simulink model "s3_PMSG"  (R2019b)
settings: Solver=daessc  StartTime=0.0  StopTime=15  MinStep=1e-4  RelTol=1
libraries: powerlib x18, powerlib_meascontrol x2, simulink_extras x1
settings Model: SimulationMode=accelerator  Creator=MAHMUD  LastModifiedBy=MAHMUD

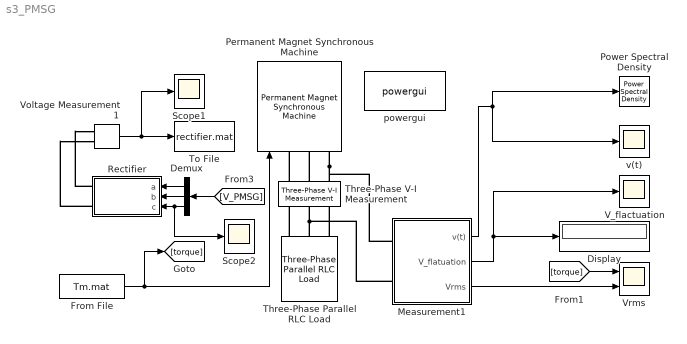
== system s3_PMSG ==
  Demux : Demux  Outputs=3
  Display : Display
  From File : FromFile  FileName=Tm.mat  SampleTime=0
  Measurement1 : Subsystem
  Permanent Magnet Synchronous Machine : powerlib/Machines/Permanent Magnet Synchronous Machine  NbPhases=3  FluxDistribution=Sinusoidal  RotorType=Salient-pole  MechanicalLoad=Torque Tm  PresetModel=No  ShowDetailedParameters=on  MeasurementBus=off  Resistance=0.03  Inductance=8.5e-3  dqInductances=[0.0415 0.015]  La=0.000835  MachineConstant=Voltage Constant (V_peak L-L / krpm)  Flux=0.55133  VoltageCst=100  TorqueCst=0.82699  Flat=120  Mechanical=[0.201 4.5 1]  PolePairs=4  InitialConditions=[0,0, 0,0]  InitialConditions5ph=[0 0 0 0 0 0]  RefAngle=Aligned with phase A axis (original Park)  IterativeDiscreteModel=Trapezoidal non iterative  TsBlock=-1  TsPowergui=0
  Power Spectral Density : simulink_extras/Additional Sinks/Power Spectral Density  npts=5000  fftpts=512  HowOften=500  sampleT=0.001
      settings: SourceProductName=Simulink  SourceProductBaseCode=SL
  Rectifier : Subsystem
  Scope1 : Scope
  Scope2 : Scope
  Three-Phase Parallel RLC Load : powerlib/Elements/Three-Phase Parallel RLC Load  LConnTagsString=A|B|C  Configuration=Y (grounded)  NominalVoltage=400  Vabc=[1e3 1e3 1e3]  Vabcp=[1e3 1e3 1e3]  NominalFrequency=50  UnbalancedPower=off  ActivePower=16e3  InductivePower=0  CapacitivePower=0  Pabc=[10e3 9e3 11e3]  QLabc=[100 90 110]  QCabc=[100 90 110]  Pabcp=[10e3 9e3 11e3]  QLabcp=[100 90 110]  QCabcp=[100 90 110]  Measurements=None  LoadType=constant Z
      settings: SourceProductName=Simscape Electrical
  Three-Phase V-I Measurement : powerlib/Measurements/Three-Phase V-I Measurement  VoltageMeasurement=phase-to-ground  SetLabelV=on  LabelV=V_PMSG  Vpu=off  VpuLL=off  CurrentMeasurement=no  SetLabelI=off  LabelI=Iabc  Ipu=off  Pbase=100e6  Vbase=500e3  OutputType=Complex  PhasorSimulation=off  PSBequivalent=0
      settings: SourceProductName=Simscape Electrical
  To File : ToFile  Filename=rectifier.mat  SaveFormat=Timeseries
  V_flactuation : Scope
  Voltage Measurement1 : powerlib/Measurements/Voltage Measurement  PhasorSimulation=off  OutputType=Complex  PSBequivalent=0
      settings: SourceProductName=Simscape Electrical
  Vrms : Scope  NumInputPorts=2
  powergui : powerlib/powergui  Priority=1  SimulationMode=Continuous  SampleTime=1e-5  frequency=60  Iterations=50  frequencyindice=0  Pbase=100e6  ErrMax=1e-4  UnitsV=kV  UnitsW=MW  buscounter=0  FunctionMessages=off  echomessages=off  EnableUseOfTLC=off  CurrentSourceSwitches=off  DisableSnubberDevices=off  DisableRonSwitches=off  DisableVfSwitches=off  DisplayEquations=off  AutomaticDiscreteSolvers=off  SolverType=Tustin/Backward Euler (TBE)  Interpol=off  ExternalGateDelay=off  methode=off  Ts=100  x0status=blocks  SPID=on  SwTol=0  HookPort=off  NonlinearTolerance=1e-4  nMaxIteration=100  ContinueOnMaxIteration=off  RestoreLinks=warning  ResistiveCurrentMeasurement=off  Frange=[0:2:500]  Ylog=off  Xlog=on  ShowGrid=off  save=off  variable=ZData  structure=0  ZoomFFT=off  StartTime=0.0  cycles=1  DisplayStyle=1  fundamental=60  FreqAxis=off  MaxFrequency=1000  frequencyindicesteady=1  RmsSteady=1  display=off
      settings: SourceProductName=Simscape Electrical
  v(t) : Scope
  wires:
  [V_PMSG] -> Demux/1
  Voltage Measurement1/1 -> Scope1/1, To File/1
  From File/1 -> Permanent Magnet Synchronous Machine/1, [torque]
  Measurement1/2(V_flatuation) -> V_flactuation/1, Display/1
  Measurement1/1(v(t)) -> v(t)/1, Power Spectral Density/1
  [torque] -> Vrms/1
  Measurement1/3(Vrms) -> Vrms/2
  Demux/1 -> Rectifier/1(a)
  Demux/2 -> Rectifier/2(b)
  Demux/3 -> Scope2/1, Rectifier/3(c)
  connections:
  Three-Phase V-I Measurement/LConn2 -- Permanent Magnet Synchronous Machine/LConn2
  Three-Phase V-I Measurement/LConn1 -- Permanent Magnet Synchronous Machine/LConn1
  Three-Phase V-I Measurement/LConn3 -- Measurement1/LConn1 -- Permanent Magnet Synchronous Machine/LConn3
  Rectifier/RConn2 -- Voltage Measurement1/LConn2
  Rectifier/RConn1 -- Voltage Measurement1/LConn1
  Three-Phase V-I Measurement/RConn2 -- Three-Phase Parallel RLC Load/LConn2 -- Measurement1/LConn2
  Three-Phase Parallel RLC Load/LConn3 -- Three-Phase V-I Measurement/RConn3
  Three-Phase Parallel RLC Load/LConn1 -- Three-Phase V-I Measurement/RConn1

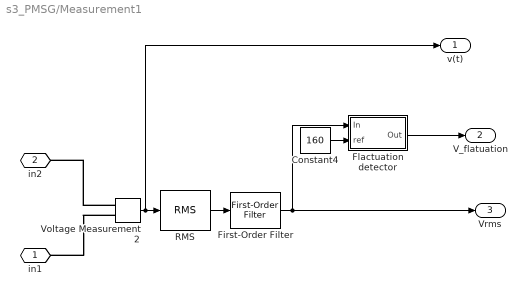
== system s3_PMSG/Measurement1 ==
  Constant4 : Constant  Value=160
  First-Order Filter : powerlib_meascontrol/Filters/First-Order Filter  FilterType=Lowpass  Tc=100e-3  Ts=0  Initialize=off  Vac_Init=[0, 0, 50]  Vdc_Init=0  PlotResponse=off  FreqRange="[0,  200,  1]"
      settings: SourceProductName=Simscape Electrical
  Flactuation detector : Subsystem
  RMS : powerlib_meascontrol/Measurements/RMS  TrueRMS=on  Freq=50  RMSInit=210  Ts=0.001
      settings: SourceProductName=Simscape Electrical
  Voltage Measurement2 : powerlib/Measurements/Voltage Measurement  PhasorSimulation=off  OutputType=Complex  PSBequivalent=0
      settings: SourceProductName=Simscape Electrical
  in1 : PMIOPort  Side=Left
  in2 : PMIOPort  Port=2  Side=Left
  v(t) : Outport
  V_flatuation : Outport  Port=2
  Vrms : Outport  Port=3
  wires:
  Voltage Measurement2/1 -> v(t)/1, RMS/1
  First-Order Filter/1 -> Vrms/1, Flactuation detector/1(In)
  RMS/1 -> First-Order Filter/1
  Flactuation detector/1(Out) -> V_flatuation/1
  Constant4/1 -> Flactuation detector/2(ref)
  connections:
  Voltage Measurement2/LConn2 -- in1/RConn1
  Voltage Measurement2/LConn1 -- in2/RConn1

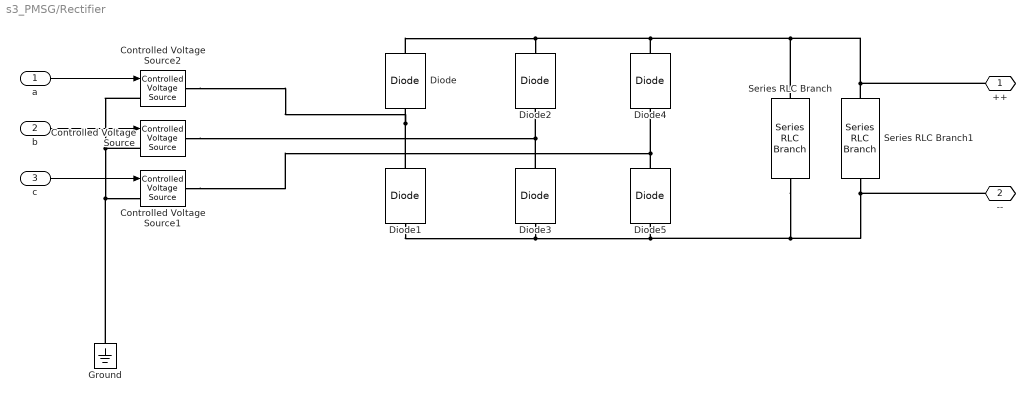
== system s3_PMSG/Rectifier ==
  a : Inport
  b : Inport  Port=2
  c : Inport  Port=3
  Controlled Voltage Source : powerlib/Electrical Sources/Controlled Voltage Source  Initialize=on  Source_Type=AC  Amplitude=0  Phase=0  Frequency=0  Measurements=None
      settings: SourceProductName=Simscape Electrical
  Controlled Voltage Source1 : powerlib/Electrical Sources/Controlled Voltage Source  Initialize=on  Source_Type=AC  Amplitude=0  Phase=0  Frequency=0  Measurements=None
      settings: SourceProductName=Simscape Electrical
  Controlled Voltage Source2 : powerlib/Electrical Sources/Controlled Voltage Source  Initialize=on  Source_Type=AC  Amplitude=0  Phase=0  Frequency=0  Measurements=None
      settings: SourceProductName=Simscape Electrical
  Diode{,1..5} (6 alike) : powerlib/Power Electronics/Diode  Ron=0.001  Lon=0  Vf=0.8  IC=0  UseSnubber=off  Rs=500  Cs=250e-9  Measurements=off
      settings: SourceProductName=Simscape Electrical
  Ground : powerlib/Elements/Ground  LConnTagsString=a
      settings: SourceProductName=Simscape Electrical
  Series RLC Branch : powerlib/Elements/Series RLC Branch  LConnTagsString=__new0  RConnTagsString=__new0  BranchType=C  Resistance=1  Inductance=1e-3  SetiL0=off  InitialCurrent=0  Capacitance=220e-6  Setx0=off  InitialVoltage=0  Measurements=None
      settings: SourceProductName=Simscape Electrical
  Series RLC Branch1 : powerlib/Elements/Series RLC Branch  LConnTagsString=__new0  RConnTagsString=__new0  BranchType=R  Resistance=10e3  Inductance=1e-3  SetiL0=off  InitialCurrent=0  Capacitance=220e-6  Setx0=off  InitialVoltage=0  Measurements=None
      settings: SourceProductName=Simscape Electrical
  ++ : PMIOPort  Side=Right
  -- : PMIOPort  Port=2  Side=Right
  wires:
  a/1 -> Controlled Voltage Source2/1
  b/1 -> Controlled Voltage Source/1
  c/1 -> Controlled Voltage Source1/1
  connections:
  Ground/LConn1 -- Controlled Voltage Source/LConn1 -- Controlled Voltage Source2/LConn1 -- Controlled Voltage Source1/LConn1
  Diode1/RConn1 -- Controlled Voltage Source2/RConn1 -- Diode/LConn1
  Diode5/RConn1 -- Controlled Voltage Source1/RConn1 -- Diode4/LConn1
  Diode1/LConn1 -- Diode3/LConn1 -- --/RConn1 -- Series RLC Branch1/RConn1 -- Series RLC Branch/RConn1 -- Diode5/LConn1
  Diode/RConn1 -- ++/RConn1 -- Series RLC Branch1/LConn1 -- Series RLC Branch/LConn1 -- Diode4/RConn1 -- Diode2/RConn1
  Diode3/RConn1 -- Controlled Voltage Source/RConn1 -- Diode2/LConn1

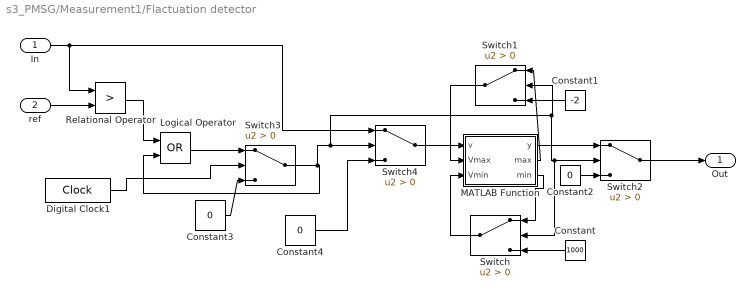
== system s3_PMSG/Measurement1/Flactuation detector ==
  In : Inport
  ref : Inport  Port=2
  Constant : Constant  Value=1000
  Constant1 : Constant  Value=-2
  Constant2 : Constant  Value=0
  Constant3 : Constant  Value=0
  Constant4 : Constant  Value=0
  Digital Clock1 : DigitalClock
  Logical Operator : Logic  Operator=OR  AllPortsSameDT=off  OutDataTypeStr=boolean
  MATLAB Function : MATLAB Function  TreatAsAtomicUnit=on
  Relational Operator : RelationalOperator  Operator=>  OutDataTypeStr=boolean  ZeroCross=off  RndMeth=Simplest
  Switch{,1..4} (5 alike) : Switch  Criteria=u2 > Threshold  ZeroCross=off
  Out : Outport
  wires:
  Constant/1 -> Switch/3
  Switch1/1 -> MATLAB Function/2(Vmax)
  Constant1/1 -> Switch1/3
  MATLAB Function/1(y) -> Switch2/1
  MATLAB Function/3(min) -> Switch/1
  Switch2/1 -> Out/1
  MATLAB Function/2(max) -> Switch1/1
  Switch/1 -> MATLAB Function/3(Vmin)
  Constant2/1 -> Switch2/3
  Logical Operator/1 -> Switch3/1
  Switch3/1 -> Switch/2, Switch2/2, Switch1/2, Switch4/2, Logical Operator/2
  Constant3/1 -> Switch3/3
  Relational Operator/1 -> Logical Operator/1
  Switch4/1 -> MATLAB Function/1(v)
  In/1 -> Relational Operator/1, Switch4/1
  Digital Clock1/1 -> Switch3/2
  ref/1 -> Relational Operator/2
  Constant4/1 -> Switch4/3

== matlab function s3_PMSG/Measurement1/Flactuation detector/MATLAB Function ==
  data: v input; y output; Vmax input; Vmin input; max output; min output
function [y,max,min] = fcn(v,Vmax,Vmin)
if(v>0)
    if(v<Vmin)
        min=v;
    else
        min=Vmin;
    end
    if(v>Vmax)
        max=v;
    else 
        max=Vmax;
    end
    y=Vmax-Vmin;
else
    min=0;
    max=0;
    y=0;
end
